simulink model "TST_AFS_DD1ms"  (R2016b)
settings: Solver=FixedStepDiscrete  StartTime=0.0  StopTime=simTime  FixedStep=sampleTime  RelTol=1e-3
values from neighbouring files (symbols this model uses):
  testCase = 1    [initTST_AFS_DD1ms_001.m]
libraries: simulink x4, UnitTest_Lib x2
settings Model: Creator=zhengjinyan  LastModifiedBy=zhengjinyan
settings DebuggingCC: SignalRangeChecking=error

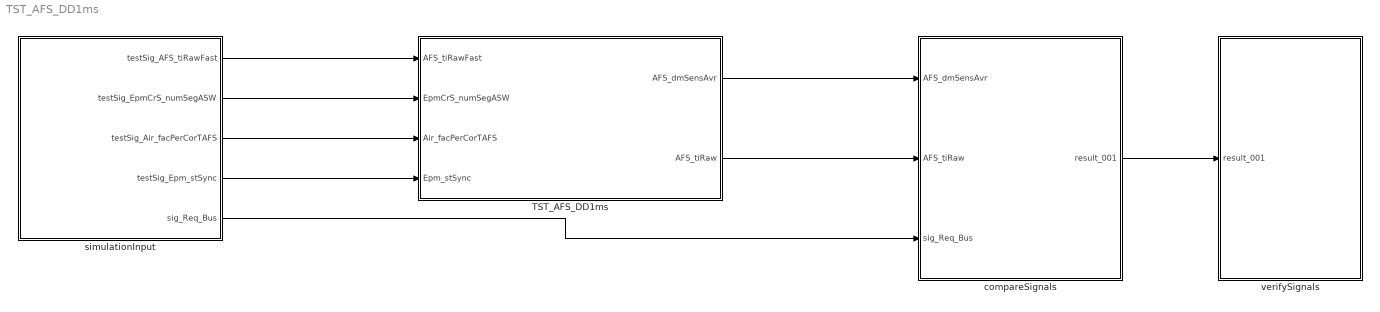
== system TST_AFS_DD1ms ==
  TST_AFS_DD1ms : Subsystem
  compareSignals : Subsystem
  simulationInput : Subsystem
  verifySignals : Subsystem
  wires:
  simulationInput/1(testSig_AFS_tiRawFast) -> TST_AFS_DD1ms/1(AFS_tiRawFast)
  simulationInput/2(testSig_EpmCrS_numSegASW) -> TST_AFS_DD1ms/2(EpmCrS_numSegASW)
  simulationInput/3(testSig_Air_facPerCorTAFS) -> TST_AFS_DD1ms/3(Air_facPerCorTAFS)
  simulationInput/4(testSig_Epm_stSync) -> TST_AFS_DD1ms/4(Epm_stSync)
  TST_AFS_DD1ms/1(AFS_dmSensAvr) -> compareSignals/1(AFS_dmSensAvr)
  TST_AFS_DD1ms/2(AFS_tiRaw) -> compareSignals/2(AFS_tiRaw)
  simulationInput/5(sig_Req_Bus) -> compareSignals/3(sig_Req_Bus)
  compareSignals/1(result_001) -> verifySignals/1(result_001)

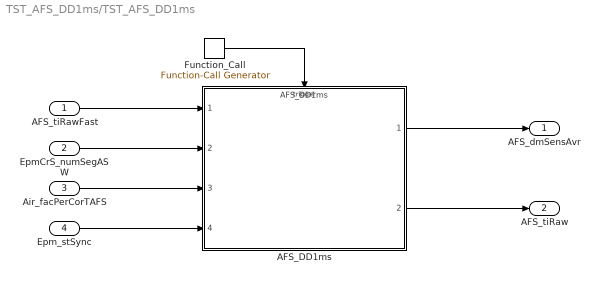
== system TST_AFS_DD1ms/TST_AFS_DD1ms ==
  AFS_tiRawFast : Inport
  EpmCrS_numSegASW : Inport  Port=2
  Air_facPerCorTAFS : Inport  Port=3
  Epm_stSync : Inport  Port=4
  AFS_DD1ms : ModelReference  ModelNameDialog=AFS_DD1ms  SimulationMode=Normal  ModelReferenceVersion=1.34  TriggerPortName=function  TriggerPortTriggerType=function-call  TriggerPortStatesWhenEnabling=held
  Function_Call : simulink/Ports & Subsystems/Function-Call Generator  sample_time=sampleTime  numberOfIterations=1
  AFS_dmSensAvr : Outport
  AFS_tiRaw : Outport  Port=2
  wires:
  Function_Call/1 -> AFS_DD1ms/Trigger
  AFS_tiRawFast/1 -> AFS_DD1ms/1
  EpmCrS_numSegASW/1 -> AFS_DD1ms/2
  Air_facPerCorTAFS/1 -> AFS_DD1ms/3
  Epm_stSync/1 -> AFS_DD1ms/4
  AFS_DD1ms/1 -> AFS_dmSensAvr/1
  AFS_DD1ms/2 -> AFS_tiRaw/1

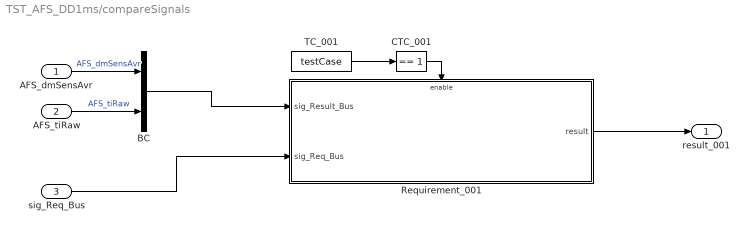
== system TST_AFS_DD1ms/compareSignals ==
  AFS_dmSensAvr : Inport
  AFS_tiRaw : Inport  Port=2
  sig_Req_Bus : Inport  Port=3
  BC : BusCreator  Inputs=2
  CTC_001 : simulink/Logic and Bit Operations/Compare To Constant  relop===  const=1  OutDataTypeStr=boolean
  Requirement_001 : Subsystem
  TC_001 : Constant  Value=testCase
  result_001 : Outport
  wires:
  AFS_dmSensAvr/1 -> BC/1  "AFS_dmSensAvr"
  AFS_tiRaw/1 -> BC/2  "AFS_tiRaw"
  TC_001/1 -> CTC_001/1
  CTC_001/1 -> Requirement_001/Enable
  sig_Req_Bus/1 -> Requirement_001/2(sig_Req_Bus)
  BC/1 -> Requirement_001/1(sig_Result_Bus)
  Requirement_001/1(result) -> result_001/1

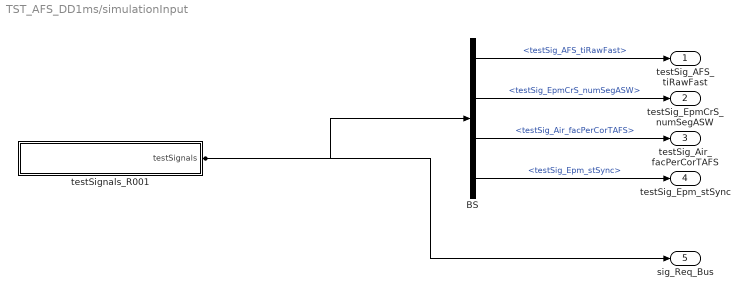
== system TST_AFS_DD1ms/simulationInput ==
  BS : BusSelector  OutputSignals=testSig_AFS_tiRawFast,testSig_EpmCrS_numSegASW,testSig_Air_facPerCorTAFS,testSig_Epm_stSync
  testSignals_R001 : Subsystem
  testSig_AFS_tiRawFast : Outport
  testSig_EpmCrS_numSegASW : Outport  Port=2
  testSig_Air_facPerCorTAFS : Outport  Port=3
  testSig_Epm_stSync : Outport  Port=4
  sig_Req_Bus : Outport  Port=5
  wires:
  BS/1 -> testSig_AFS_tiRawFast/1  "<testSig_AFS_tiRawFast>"
  BS/2 -> testSig_EpmCrS_numSegASW/1  "<testSig_EpmCrS_numSegASW>"
  BS/3 -> testSig_Air_facPerCorTAFS/1  "<testSig_Air_facPerCorTAFS>"
  BS/4 -> testSig_Epm_stSync/1  "<testSig_Epm_stSync>"
  testSignals_R001/1(testSignals) -> BS/1, sig_Req_Bus/1

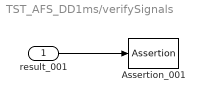
== system TST_AFS_DD1ms/verifySignals ==
  result_001 : Inport
  Assertion_001 : Assertion  Enabled=off
  wires:
  result_001/1 -> Assertion_001/1

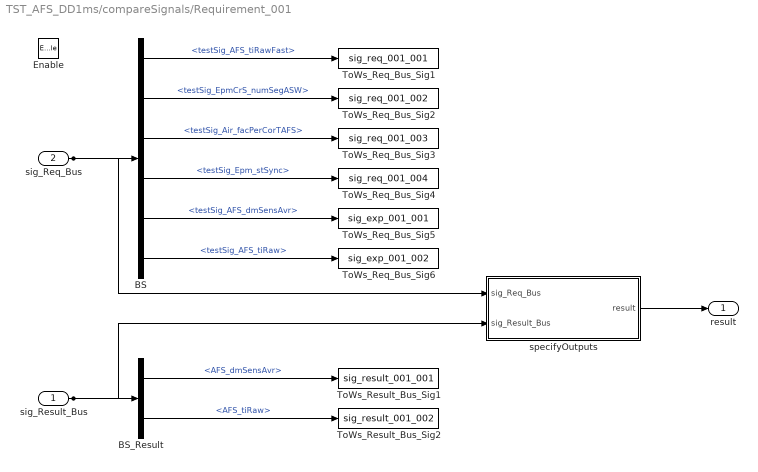
== system TST_AFS_DD1ms/compareSignals/Requirement_001 ==
  sig_Result_Bus : Inport
  sig_Req_Bus : Inport  Port=2
  Enable : EnablePort
  BS : BusSelector  OutputSignals=testSig_AFS_tiRawFast,testSig_EpmCrS_numSegASW,testSig_Air_facPerCorTAFS,testSig_Epm_stSync,testSig_AFS_dmSensAvr,testSig_AFS_tiRaw
  BS_Result : BusSelector  OutputSignals=AFS_dmSensAvr,AFS_tiRaw
  ToWs_Req_Bus_Sig1 : ToWorkspace  VariableName=sig_req_001_001  SaveFormat=Structure With Time
  ToWs_Req_Bus_Sig2 : ToWorkspace  VariableName=sig_req_001_002  SaveFormat=Structure With Time
  ToWs_Req_Bus_Sig3 : ToWorkspace  VariableName=sig_req_001_003  SaveFormat=Structure With Time
  ToWs_Req_Bus_Sig4 : ToWorkspace  VariableName=sig_req_001_004  SaveFormat=Structure With Time
  ToWs_Req_Bus_Sig5 : ToWorkspace  VariableName=sig_exp_001_001  SaveFormat=Structure With Time
  ToWs_Req_Bus_Sig6 : ToWorkspace  VariableName=sig_exp_001_002  SaveFormat=Structure With Time
  ToWs_Result_Bus_Sig1 : ToWorkspace  VariableName=sig_result_001_001  SaveFormat=Structure With Time
  ToWs_Result_Bus_Sig2 : ToWorkspace  VariableName=sig_result_001_002  SaveFormat=Structure With Time
  specifyOutputs : Subsystem
  result : Outport
  wires:
  sig_Req_Bus/1 -> BS/1, specifyOutputs/1(sig_Req_Bus)
  BS/1 -> ToWs_Req_Bus_Sig1/1  "<testSig_AFS_tiRawFast>"
  BS/2 -> ToWs_Req_Bus_Sig2/1  "<testSig_EpmCrS_numSegASW>"
  BS/3 -> ToWs_Req_Bus_Sig3/1  "<testSig_Air_facPerCorTAFS>"
  BS/4 -> ToWs_Req_Bus_Sig4/1  "<testSig_Epm_stSync>"
  BS/5 -> ToWs_Req_Bus_Sig5/1  "<testSig_AFS_dmSensAvr>"
  BS/6 -> ToWs_Req_Bus_Sig6/1  "<testSig_AFS_tiRaw>"
  sig_Result_Bus/1 -> BS_Result/1, specifyOutputs/2(sig_Result_Bus)
  BS_Result/1 -> ToWs_Result_Bus_Sig1/1  "<AFS_dmSensAvr>"
  BS_Result/2 -> ToWs_Result_Bus_Sig2/1  "<AFS_tiRaw>"
  specifyOutputs/1(result) -> result/1

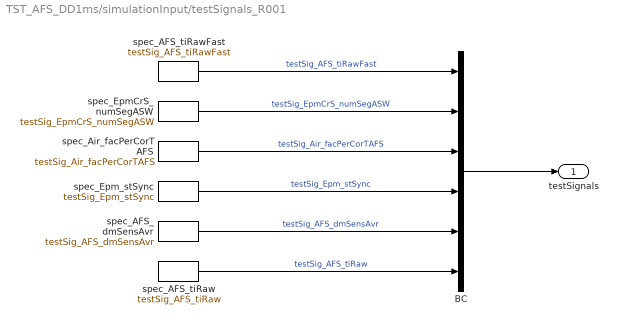
== system TST_AFS_DD1ms/simulationInput/testSignals_R001 ==
  BC : BusCreator  Inputs=6
  spec_AFS_dmSensAvr : FromWorkspace  VariableName=testSig_AFS_dmSensAvr  Interpolate=off  OutputAfterFinalValue=Holding final value
  spec_AFS_tiRaw : FromWorkspace  VariableName=testSig_AFS_tiRaw  Interpolate=off  OutputAfterFinalValue=Holding final value
  spec_AFS_tiRawFast : FromWorkspace  VariableName=testSig_AFS_tiRawFast  Interpolate=off  OutputAfterFinalValue=Holding final value
  spec_Air_facPerCorTAFS : FromWorkspace  VariableName=testSig_Air_facPerCorTAFS  Interpolate=off  OutputAfterFinalValue=Holding final value
  spec_EpmCrS_numSegASW : FromWorkspace  VariableName=testSig_EpmCrS_numSegASW  Interpolate=off  OutputAfterFinalValue=Holding final value
  spec_Epm_stSync : FromWorkspace  VariableName=testSig_Epm_stSync  Interpolate=off  OutputAfterFinalValue=Holding final value
  testSignals : Outport
  wires:
  BC/1 -> testSignals/1
  spec_AFS_tiRawFast/1 -> BC/1  "testSig_AFS_tiRawFast"
  spec_EpmCrS_numSegASW/1 -> BC/2  "testSig_EpmCrS_numSegASW"
  spec_Air_facPerCorTAFS/1 -> BC/3  "testSig_Air_facPerCorTAFS"
  spec_Epm_stSync/1 -> BC/4  "testSig_Epm_stSync"
  spec_AFS_dmSensAvr/1 -> BC/5  "testSig_AFS_dmSensAvr"
  spec_AFS_tiRaw/1 -> BC/6  "testSig_AFS_tiRaw"

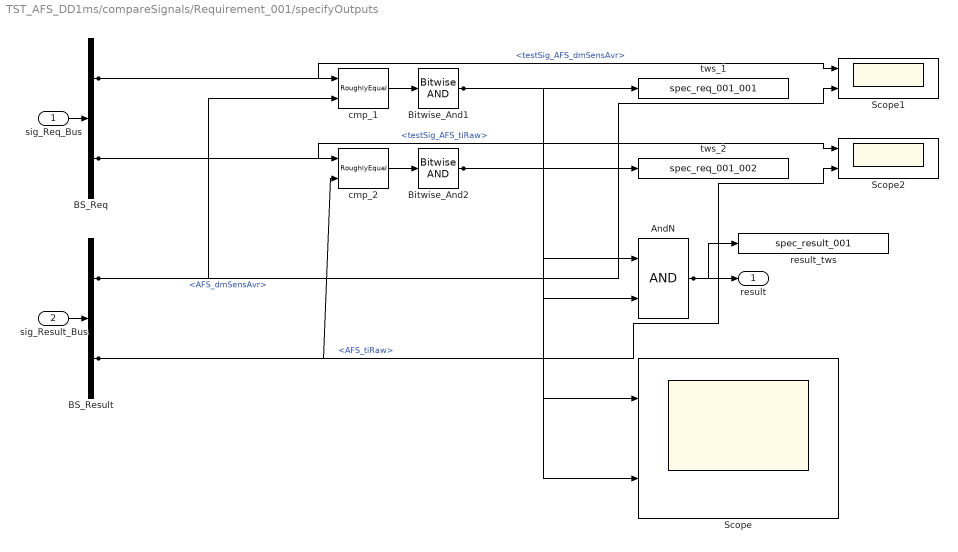
== system TST_AFS_DD1ms/compareSignals/Requirement_001/specifyOutputs ==
  sig_Req_Bus : Inport
  sig_Result_Bus : Inport  Port=2
  AndN : Logic
  BS_Req : BusSelector  OutputSignals=testSig_AFS_dmSensAvr,testSig_AFS_tiRaw
  BS_Result : BusSelector  OutputSignals=AFS_dmSensAvr,AFS_tiRaw
  Bitwise_And1 : simulink/Logic and Bit Operations/Bitwise Operator  logicop=AND  UseBitMask=off  BitMask=bin2dec('11011001')  BitMaskRealWorld=Stored Integer
  Bitwise_And2 : simulink/Logic and Bit Operations/Bitwise Operator  logicop=AND  UseBitMask=off  BitMask=bin2dec('11011001')  BitMaskRealWorld=Stored Integer
  Scope : Scope  NumInputPorts=2
  Scope1 : Scope  NumInputPorts=2
  Scope2 : Scope  NumInputPorts=2
  cmp_1 : UnitTest_Lib/RoughlyEqual  slope=0.1
  cmp_2 : UnitTest_Lib/RoughlyEqual  slope=0.1
  result_tws : ToWorkspace  VariableName=spec_result_001
  tws_1 : ToWorkspace  VariableName=spec_req_001_001
  tws_2 : ToWorkspace  VariableName=spec_req_001_002
  result : Outport
  wires:
  sig_Req_Bus/1 -> BS_Req/1
  sig_Result_Bus/1 -> BS_Result/1
  AndN/1 -> result/1, result_tws/1
  BS_Req/1 -> cmp_1/1, Scope1/1  "<testSig_AFS_dmSensAvr>"
  BS_Result/1 -> cmp_1/2, Scope1/2  "<AFS_dmSensAvr>"
  cmp_1/1 -> Bitwise_And1/1
  Bitwise_And1/1 -> tws_1/1, AndN/1, Scope/1
  BS_Req/2 -> cmp_2/1, Scope2/1  "<testSig_AFS_tiRaw>"
  BS_Result/2 -> cmp_2/2, Scope2/2  "<AFS_tiRaw>"
  cmp_2/1 -> Bitwise_And2/1
  Bitwise_And2/1 -> tws_2/1, AndN/2, Scope/2
